simulink model "proj_sub"  (R2022b)
settings: Solver=VariableStepAuto  StartTime=0.0  StopTime=10.0  RelTol=1e-3
undefined symbols (not defined in the file): a, b, c, DiscIntNeverNeededParam
libraries: hdlsllib x6, slpidlib x4, dspswit3 x1
settings Model: Creator=fadii  LastModifiedBy=fadii

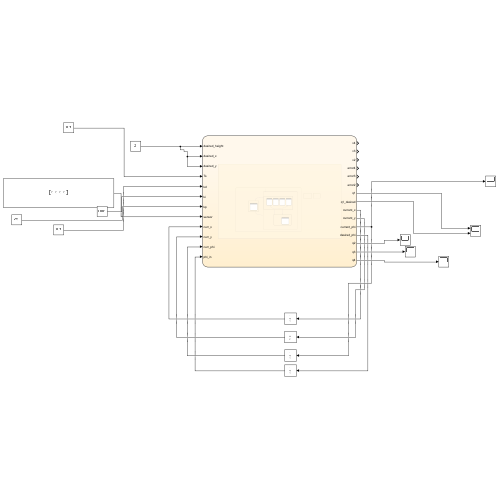
[thumbnail: Simulink's stored preview of the top-level diagram]
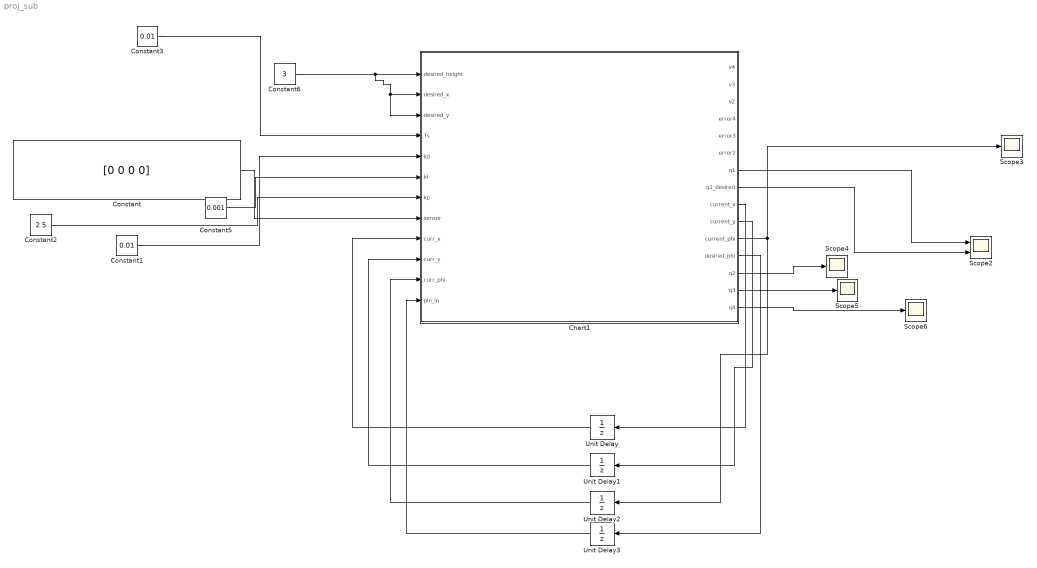
== system proj_sub ==
  Chart1 : Stateflow chart  TreatAsAtomicUnit=on
  Constant : Constant  Value=[0 0 0 0]
  Constant1 : Constant  Value=0.01
  Constant2 : Constant  Value=2.5
  Constant3 : Constant  Value=0.01
  Constant5 : Constant  Value=0.001
  Constant6 : Constant  Value=3
  Scope2 : Scope  NumInputPorts=2
  Scope{3..6} (4 alike) : Scope
  Unit Delay{,1..3} (4 alike) : UnitDelay  SampleTime=-1  HasFrameUpgradeWarning=on
  wires:
  Chart1/13(q2) -> Scope4/1
  Unit Delay1/1 -> Chart1/10(curr_y)
  Chart1/10(current_y) -> Unit Delay1/1
  Unit Delay2/1 -> Chart1/11(curr_phi)
  Constant6/1 -> Chart1/3(desired_y), Chart1/2(desired_x), Chart1/1(desired_height)
  Constant2/1 -> Chart1/7(kp)
  Constant3/1 -> Chart1/4(Ts)
  Chart1/14(q3) -> Scope5/1
  Chart1/12(desired_phi) -> Unit Delay3/1
  Chart1/11(current_phi) -> Scope3/1, Unit Delay2/1
  Chart1/8(q1_desired) -> Scope2/2
  Chart1/9(current_x) -> Unit Delay/1
  Constant1/1 -> Chart1/5(kd)
  Unit Delay3/1 -> Chart1/12(phi_in)
  Chart1/15(q4) -> Scope6/1
  Chart1/7(q1) -> Scope2/1
  Unit Delay/1 -> Chart1/9(curr_x)
  Constant/1 -> Chart1/8(sensor)
  Constant5/1 -> Chart1/6(ki)

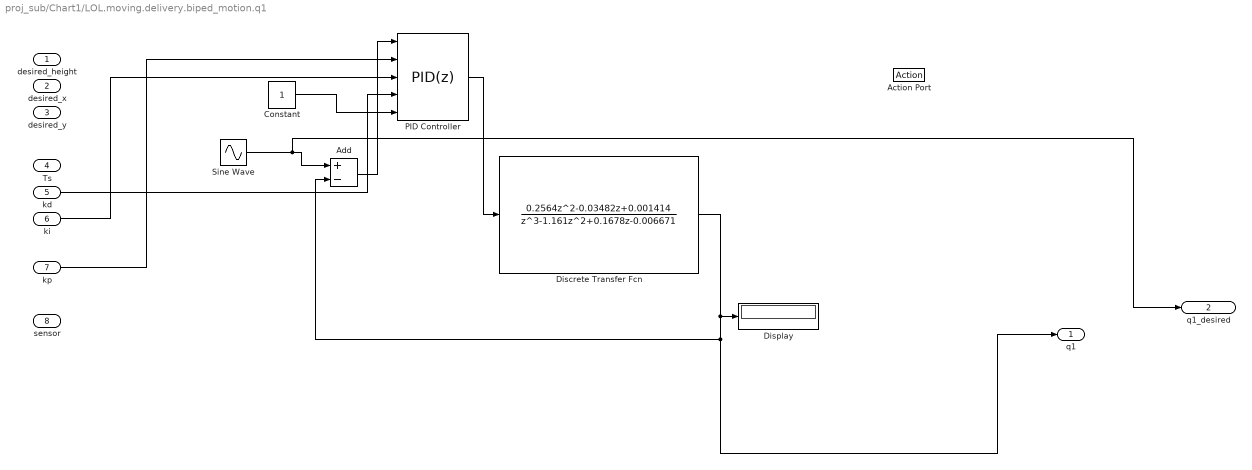
== system proj_sub/Chart1/LOL.moving.delivery.biped_motion.q1 ==
  desired_height : Inport
  desired_x : Inport  Port=2
  desired_y : Inport  Port=3
  Ts : Inport  Port=4
  kd : Inport  Port=5
  ki : Inport  Port=6
  kp : Inport  Port=7
  sensor : Inport  Port=8
  Action Port : ActionPort
      settings: CopyFcn=Stateflow.SLINSF.SimulinkMan.removeBlockPreDeleteFcn  PreDeleteFcn=Stateflow.SLINSF.SimulinkMan.unsafePredeleteFcn
  Add : Sum  Inputs=+-
  Constant : Constant
  Discrete Transfer Fcn : DiscreteTransferFcn  Numerator=[0 0.2564 -0.03482 0.001414]  Denominator=[1 -1.161 0.1678 -0.006671]  SampleTime=0.1
  Display : Display
  PID Controller : slpidlib/PID Controller  Controller=PID  Form=Parallel  TimeDomain=Discrete-time  UseExternalTs=off  SampleTime=0.1  IntegratorMethod=Forward Euler  FilterMethod=Forward Euler  ControllerParametersSource=external  P=1  I=0.002  UseKiTs=off  D=0.01  N=100  UseFilter=on  TunerSelectOption=Transfer Function Based (PID Tuner App)  InitialConditionSource=internal  InitialConditionForIntegrator=0  InitialConditionForFilter=0  DifferentiatorICPrevScaledInput=0  ExternalReset=none  TrackingMode=off  Kt=1  LimitOutput=on  SatLimitsSource=internal  UpperSaturationLimit=24  LowerSaturationLimit=-24  LinearizeAsGain=on  AntiWindupMode=none  Kb=1  LimitIntegrator=off  UpperIntegratorSaturationLimit=inf  LowerIntegratorSaturationLimit=-inf  POutMin=[]  POutMax=[]  IOutMin=[]  IOutMax=[]  DOutMin=[]  DOutMax=[]  NOutMin=[]  NOutMax=[]  SumOutMin=[]  SumOutMax=[]  SaturationOutMin=[]  SaturationOutMax=[]  PParamMin=[]  PParamMax=[]  IParamMin=[]  IParamMax=[]  DParamMin=[]  DParamMax=[]  NParamMin=[]  NParamMax=[]  KbParamMin=[]  KbParamMax=[]  KtParamMin=[]  KtParamMax=[]  KbOutMin=[]  KbOutMax=[]  KtOutMin=[]  KtOutMax=[]  IntegratorOutMin=[]  IntegratorOutMax=[]  FilterOutMin=[]  FilterOutMax=[]  SumI1OutMin=[]  SumI1OutMax=[]  SumI2OutMin=[]  SumI2OutMax=[]  SumI3OutMin=[]  SumI3OutMax=[]  SumI4OutMin=[]  SumI4OutMax=[]  SumDOutMin=[]  SumDOutMax=[]  DifferentiatorOutMin=[]  DifferentiatorOutMax=[]  FilterDiffOutCoefMin=[]  FilterDiffOutCoefMax=[]  ReciprocalOutMin=[]  ReciprocalOutMax=[]  SumDenOutMin=[]  SumDenOutMax=[]  SumNumOutMin=[]  SumNumOutMax=[]  DivideOutMin=[]  DivideOutMax=[]  UdiffTsProdOutMin=[]  UdiffTsProdOutMax=[]  NTsProdOutMin=[]  NTsProdOutMax=[]  UintegralTsProdOutMin=[]  UintegralTsProdOutMax=[]  UngainTsProdOutMin=[]  UngainTsProdOutMax=[]  ClampingZeroOutDataTypeStr=Inherit: Inherit via back propagation  ClampingZeroOutMin=[]  ClampingZeroOutMax=[]  FilterDenConstantOutDataTypeStr=Inherit: Inherit via back propagation  FilterDenConstantOutMin=[]  FilterDenConstantOutMax=[]  PCopyOutDataTypeStr=Inherit: Inherit via back propagation  PCopyOutMin=[]  PCopyOutMax=[]  NCopyOutDataTypeStr=Inherit: Inherit via back propagation  NCopyOutMin=[]  NCopyOutMax=[]  IntegratorContinuousStateAttributes=''  IntegratorStateMustResolveToSignalObject=off  IntegratorRTWStateStorageClass=Auto  FilterContinuousStateAttributes=''  FilterStateMustResolveToSignalObject=off  FilterRTWStateStorageClass=Auto  ParallelPVariant=ExternalParameters  IdealPVariant=Disabled  IVariant=ExternalParameters  DVariant=ExternalParameters  IntegratorVariant=Discrete  SatVariant=Enabled  AWVariant=Passthrough  PCopyVariant=Disabled  TRVariant=Disabled  FdbkBlocksVariant=Forward  IdealPFdbkVariant=Disabled  SatFdbkVariant=Disabled  DerivativeFilterVariant=ForwardEulerFilter  NVariant=ExternalParameters  NCopyVariant=Disabled  FilterICVariant=InternalICsFilter  IntegratorICVariant=InternalICs  ExternalResetVariant=Disabled  TRSumVariant=Passthrough  SumFdbkVariant=Disabled  SumVariant=Sum_PID  TsampFilterVariant=InternalTs  TsampNgainVariant=Passthrough  TsampIntegralVariant=Passthrough  ExternalSaturationOutDataTypeStr=Inherit: Same as second input
  Sine Wave : Sin  SineType=Sample based  Amplitude=20*pi/180  SampleTime=0.1
  q1 : Outport
  q1_desired : Outport  Port=2
  wires:
  Sine Wave/1 -> q1_desired/1, Add/1
  Add/1 -> PID Controller/1
  PID Controller/1 -> Discrete Transfer Fcn/1
  Discrete Transfer Fcn/1 -> q1/1, Add/2, Display/1
  Constant/1 -> PID Controller/5
  kp/1 -> PID Controller/2
  ki/1 -> PID Controller/3
  kd/1 -> PID Controller/4

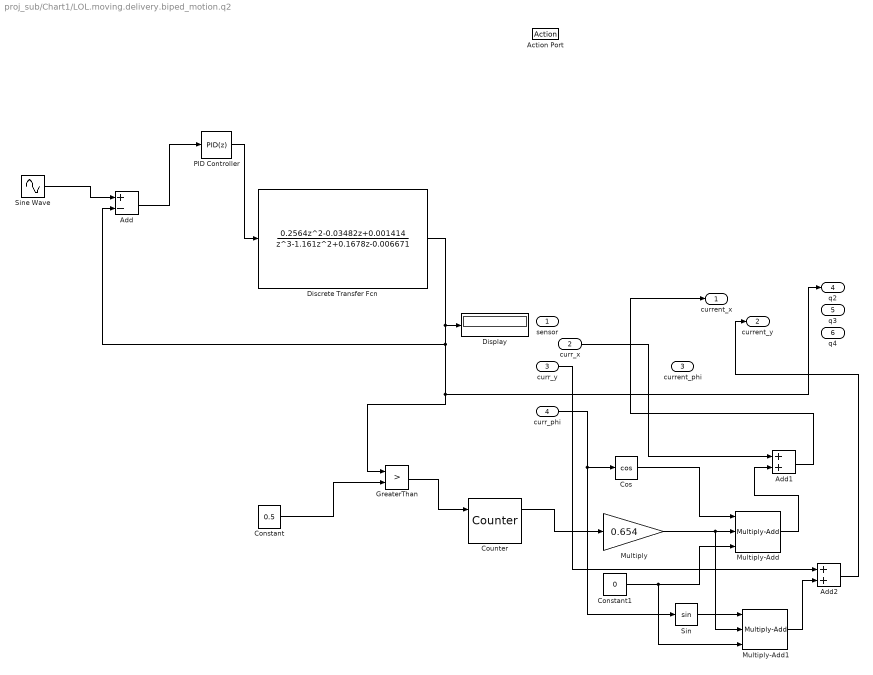
== system proj_sub/Chart1/LOL.moving.delivery.biped_motion.q2 ==
  sensor : Inport
  curr_x : Inport  Port=2
  curr_y : Inport  Port=3
  curr_phi : Inport  Port=4
  Action Port : ActionPort
      settings: CopyFcn=Stateflow.SLINSF.SimulinkMan.removeBlockPreDeleteFcn  PreDeleteFcn=Stateflow.SLINSF.SimulinkMan.unsafePredeleteFcn
  Add : Sum  Inputs=+-
  Add1 : Sum
  Add2 : Sum
  Constant : Constant  Value=0.5
  Constant1 : Constant  Value=0
  Cos : Trigonometry  Operator=cos
  Counter : dspswit3/Counter  Direction=Up  CountEvent=Rising edge  CounterSize=User defined  MaxCount=1024  InitialCount=0  Output=Count and Hit  HitValue=32  ResetInput=on  SamplesPerFrame=1  Ts=1  CntDtype=double  HitDtype=Logical
  Discrete Transfer Fcn : DiscreteTransferFcn  Numerator=[0 0.2564 -0.03482 0.001414]  Denominator=[1 -1.161 0.1678 -0.006671]  SampleTime=0.1
  Display : Display
  GreaterThan : RelationalOperator  Operator=>  OutDataTypeStr=boolean  RndMeth=Simplest  InputSameDT=off
  Multiply : Gain  Gain=0.654
  Multiply-Add : hdlsllib/HDL Operations/Multiply-Add  Function=c+(a.*b)  datatype=Inherit: Inherit via internal rule  DoSatur=off  FMA=off
  Multiply-Add1 : hdlsllib/HDL Operations/Multiply-Add  Function=c+(a.*b)  datatype=Inherit: Inherit via internal rule  DoSatur=off  FMA=off
  PID Controller : slpidlib/PID Controller  Controller=PID  Form=Parallel  TimeDomain=Discrete-time  UseExternalTs=off  SampleTime=0.1  IntegratorMethod=Forward Euler  FilterMethod=Forward Euler  ControllerParametersSource=internal  P=1  I=1  UseKiTs=off  D=0  N=100  UseFilter=on  TunerSelectOption=Transfer Function Based (PID Tuner App)  InitialConditionSource=internal  InitialConditionForIntegrator=0  InitialConditionForFilter=0  DifferentiatorICPrevScaledInput=0  ExternalReset=none  TrackingMode=off  Kt=1  LimitOutput=off  SatLimitsSource=internal  UpperSaturationLimit=inf  LowerSaturationLimit=-inf  LinearizeAsGain=on  AntiWindupMode=none  Kb=1  LimitIntegrator=off  UpperIntegratorSaturationLimit=inf  LowerIntegratorSaturationLimit=-inf  POutMin=[]  POutMax=[]  IOutMin=[]  IOutMax=[]  DOutMin=[]  DOutMax=[]  NOutMin=[]  NOutMax=[]  SumOutMin=[]  SumOutMax=[]  SaturationOutMin=[]  SaturationOutMax=[]  PParamMin=[]  PParamMax=[]  IParamMin=[]  IParamMax=[]  DParamMin=[]  DParamMax=[]  NParamMin=[]  NParamMax=[]  KbParamMin=[]  KbParamMax=[]  KtParamMin=[]  KtParamMax=[]  KbOutMin=[]  KbOutMax=[]  KtOutMin=[]  KtOutMax=[]  IntegratorOutMin=[]  IntegratorOutMax=[]  FilterOutMin=[]  FilterOutMax=[]  SumI1OutMin=[]  SumI1OutMax=[]  SumI2OutMin=[]  SumI2OutMax=[]  SumI3OutMin=[]  SumI3OutMax=[]  SumI4OutMin=[]  SumI4OutMax=[]  SumDOutMin=[]  SumDOutMax=[]  DifferentiatorOutMin=[]  DifferentiatorOutMax=[]  FilterDiffOutCoefMin=[]  FilterDiffOutCoefMax=[]  ReciprocalOutMin=[]  ReciprocalOutMax=[]  SumDenOutMin=[]  SumDenOutMax=[]  SumNumOutMin=[]  SumNumOutMax=[]  DivideOutMin=[]  DivideOutMax=[]  UdiffTsProdOutMin=[]  UdiffTsProdOutMax=[]  NTsProdOutMin=[]  NTsProdOutMax=[]  UintegralTsProdOutMin=[]  UintegralTsProdOutMax=[]  UngainTsProdOutMin=[]  UngainTsProdOutMax=[]  ClampingZeroOutDataTypeStr=Inherit: Inherit via back propagation  ClampingZeroOutMin=[]  ClampingZeroOutMax=[]  FilterDenConstantOutDataTypeStr=Inherit: Inherit via back propagation  FilterDenConstantOutMin=[]  FilterDenConstantOutMax=[]  PCopyOutDataTypeStr=Inherit: Inherit via back propagation  PCopyOutMin=[]  PCopyOutMax=[]  NCopyOutDataTypeStr=Inherit: Inherit via back propagation  NCopyOutMin=[]  NCopyOutMax=[]  IntegratorContinuousStateAttributes=''  IntegratorStateMustResolveToSignalObject=off  IntegratorRTWStateStorageClass=Auto  FilterContinuousStateAttributes=''  FilterStateMustResolveToSignalObject=off  FilterRTWStateStorageClass=Auto  ParallelPVariant=InternalParameters  IdealPVariant=Disabled  IVariant=InternalParameters  DVariant=InternalParameters  IntegratorVariant=Discrete  SatVariant=Disabled  AWVariant=Passthrough  PCopyVariant=Disabled  TRVariant=Disabled  FdbkBlocksVariant=Forward  IdealPFdbkVariant=Disabled  SatFdbkVariant=Disabled  DerivativeFilterVariant=ForwardEulerFilter  NVariant=InternalParameters  NCopyVariant=Disabled  FilterICVariant=InternalICsFilter  IntegratorICVariant=InternalICs  ExternalResetVariant=Disabled  TRSumVariant=Passthrough  SumFdbkVariant=Disabled  SumVariant=Sum_PID  TsampFilterVariant=InternalTs  TsampNgainVariant=Passthrough  TsampIntegralVariant=Passthrough  ExternalSaturationOutDataTypeStr=Inherit: Same as second input
  Sin : Trigonometry
  Sine Wave : Sin  SineType=Sample based  Amplitude=30*pi/180  Bias=30*pi/180  SampleTime=0.1  Offset=2
  current_x : Outport
  current_y : Outport  Port=2
  current_phi : Outport  Port=3
  q2 : Outport  Port=4
  q3 : Outport  Port=5
  q4 : Outport  Port=6
  wires:
  Constant/1 -> GreaterThan/2
  GreaterThan/1 -> Counter/1
  Add/1 -> PID Controller/1
  Discrete Transfer Fcn/1 -> GreaterThan/1, q2/1, Add/2, Display/1
  PID Controller/1 -> Discrete Transfer Fcn/1
  Sine Wave/1 -> Add/1
  Counter/1 -> Multiply/1
  curr_phi/1 -> Sin/1, Cos/1
  curr_x/1 -> Add1/1
  Add1/1 -> current_x/1
  Constant1/1 -> Multiply-Add1/3, Multiply-Add/3
  Multiply/1 -> Multiply-Add1/2, Multiply-Add/2
  Cos/1 -> Multiply-Add/1
  Multiply-Add/1 -> Add1/2
  Sin/1 -> Multiply-Add1/1
  Multiply-Add1/1 -> Add2/2
  curr_y/1 -> Add2/1
  Add2/1 -> current_y/1

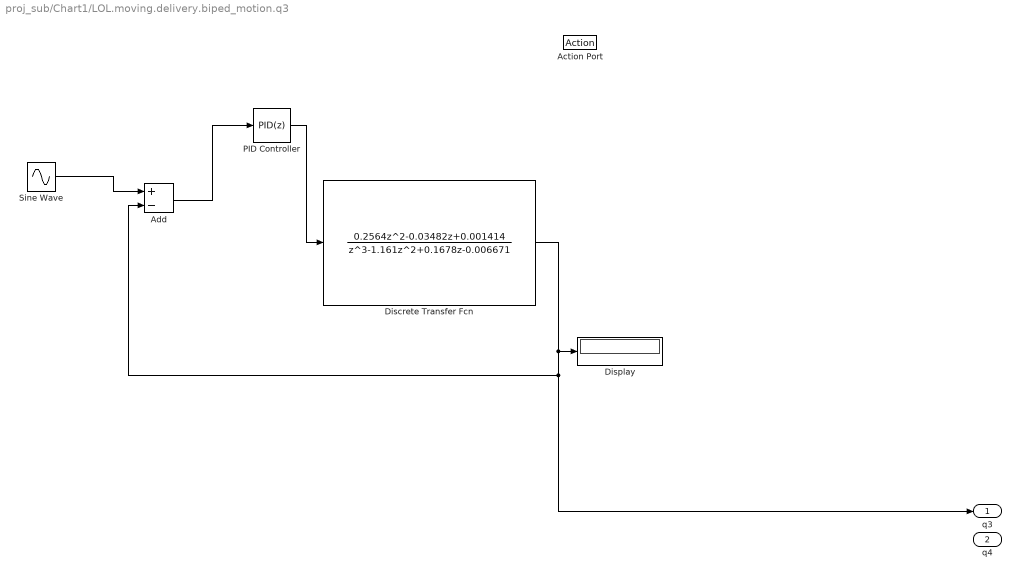
== system proj_sub/Chart1/LOL.moving.delivery.biped_motion.q3 ==
  Action Port : ActionPort
      settings: CopyFcn=Stateflow.SLINSF.SimulinkMan.removeBlockPreDeleteFcn  PreDeleteFcn=Stateflow.SLINSF.SimulinkMan.unsafePredeleteFcn
  Add : Sum  Inputs=+-
  Discrete Transfer Fcn : DiscreteTransferFcn  Numerator=[0 0.2564 -0.03482 0.001414]  Denominator=[1 -1.161 0.1678 -0.006671]  SampleTime=0.1
  Display : Display
  PID Controller : slpidlib/PID Controller  Controller=PID  Form=Parallel  TimeDomain=Discrete-time  UseExternalTs=off  SampleTime=0.1  IntegratorMethod=Forward Euler  FilterMethod=Forward Euler  ControllerParametersSource=internal  P=1  I=1  UseKiTs=off  D=0  N=100  UseFilter=on  TunerSelectOption=Transfer Function Based (PID Tuner App)  InitialConditionSource=internal  InitialConditionForIntegrator=0  InitialConditionForFilter=0  DifferentiatorICPrevScaledInput=0  ExternalReset=none  TrackingMode=off  Kt=1  LimitOutput=off  SatLimitsSource=internal  UpperSaturationLimit=inf  LowerSaturationLimit=-inf  LinearizeAsGain=on  AntiWindupMode=none  Kb=1  LimitIntegrator=off  UpperIntegratorSaturationLimit=inf  LowerIntegratorSaturationLimit=-inf  POutMin=[]  POutMax=[]  IOutMin=[]  IOutMax=[]  DOutMin=[]  DOutMax=[]  NOutMin=[]  NOutMax=[]  SumOutMin=[]  SumOutMax=[]  SaturationOutMin=[]  SaturationOutMax=[]  PParamMin=[]  PParamMax=[]  IParamMin=[]  IParamMax=[]  DParamMin=[]  DParamMax=[]  NParamMin=[]  NParamMax=[]  KbParamMin=[]  KbParamMax=[]  KtParamMin=[]  KtParamMax=[]  KbOutMin=[]  KbOutMax=[]  KtOutMin=[]  KtOutMax=[]  IntegratorOutMin=[]  IntegratorOutMax=[]  FilterOutMin=[]  FilterOutMax=[]  SumI1OutMin=[]  SumI1OutMax=[]  SumI2OutMin=[]  SumI2OutMax=[]  SumI3OutMin=[]  SumI3OutMax=[]  SumI4OutMin=[]  SumI4OutMax=[]  SumDOutMin=[]  SumDOutMax=[]  DifferentiatorOutMin=[]  DifferentiatorOutMax=[]  FilterDiffOutCoefMin=[]  FilterDiffOutCoefMax=[]  ReciprocalOutMin=[]  ReciprocalOutMax=[]  SumDenOutMin=[]  SumDenOutMax=[]  SumNumOutMin=[]  SumNumOutMax=[]  DivideOutMin=[]  DivideOutMax=[]  UdiffTsProdOutMin=[]  UdiffTsProdOutMax=[]  NTsProdOutMin=[]  NTsProdOutMax=[]  UintegralTsProdOutMin=[]  UintegralTsProdOutMax=[]  UngainTsProdOutMin=[]  UngainTsProdOutMax=[]  ClampingZeroOutDataTypeStr=Inherit: Inherit via back propagation  ClampingZeroOutMin=[]  ClampingZeroOutMax=[]  FilterDenConstantOutDataTypeStr=Inherit: Inherit via back propagation  FilterDenConstantOutMin=[]  FilterDenConstantOutMax=[]  PCopyOutDataTypeStr=Inherit: Inherit via back propagation  PCopyOutMin=[]  PCopyOutMax=[]  NCopyOutDataTypeStr=Inherit: Inherit via back propagation  NCopyOutMin=[]  NCopyOutMax=[]  IntegratorContinuousStateAttributes=''  IntegratorStateMustResolveToSignalObject=off  IntegratorRTWStateStorageClass=Auto  FilterContinuousStateAttributes=''  FilterStateMustResolveToSignalObject=off  FilterRTWStateStorageClass=Auto  ParallelPVariant=InternalParameters  IdealPVariant=Disabled  IVariant=InternalParameters  DVariant=InternalParameters  IntegratorVariant=Discrete  SatVariant=Disabled  AWVariant=Passthrough  PCopyVariant=Disabled  TRVariant=Disabled  FdbkBlocksVariant=Forward  IdealPFdbkVariant=Disabled  SatFdbkVariant=Disabled  DerivativeFilterVariant=ForwardEulerFilter  NVariant=InternalParameters  NCopyVariant=Disabled  FilterICVariant=InternalICsFilter  IntegratorICVariant=InternalICs  ExternalResetVariant=Disabled  TRSumVariant=Passthrough  SumFdbkVariant=Disabled  SumVariant=Sum_PID  TsampFilterVariant=InternalTs  TsampNgainVariant=Passthrough  TsampIntegralVariant=Passthrough  ExternalSaturationOutDataTypeStr=Inherit: Same as second input
  Sine Wave : Sin  SineType=Sample based  Amplitude=20*pi/180  SampleTime=0.1  Offset=10
  q3 : Outport
  q4 : Outport  Port=2
  wires:
  Sine Wave/1 -> Add/1
  Add/1 -> PID Controller/1
  PID Controller/1 -> Discrete Transfer Fcn/1
  Discrete Transfer Fcn/1 -> q3/1, Add/2, Display/1

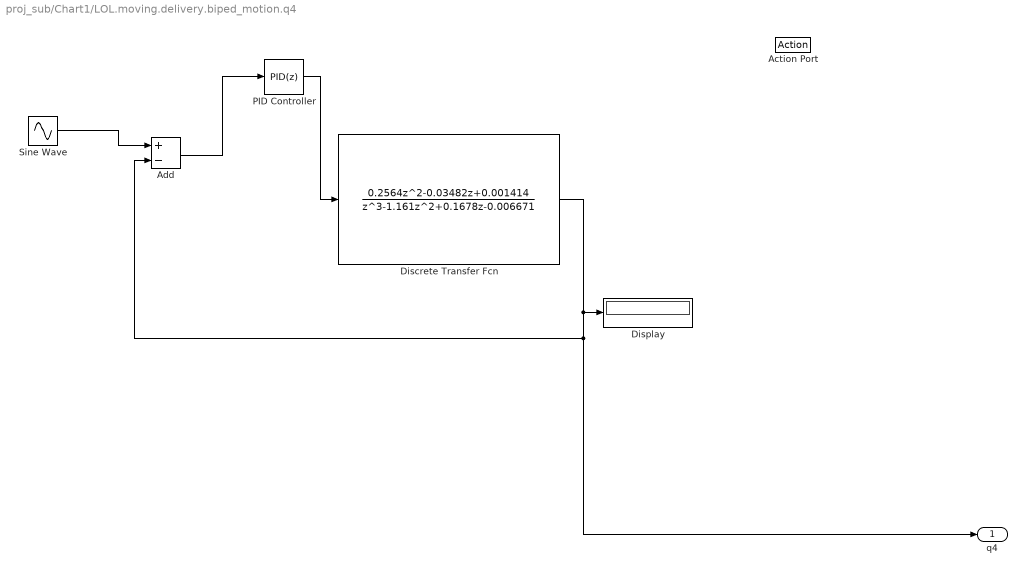
== system proj_sub/Chart1/LOL.moving.delivery.biped_motion.q4 ==
  Action Port : ActionPort
      settings: CopyFcn=Stateflow.SLINSF.SimulinkMan.removeBlockPreDeleteFcn  PreDeleteFcn=Stateflow.SLINSF.SimulinkMan.unsafePredeleteFcn
  Add : Sum  Inputs=+-
  Discrete Transfer Fcn : DiscreteTransferFcn  Numerator=[0 0.2564 -0.03482 0.001414]  Denominator=[1 -1.161 0.1678 -0.006671]  SampleTime=0.1
  Display : Display
  PID Controller : slpidlib/PID Controller  Controller=PID  Form=Parallel  TimeDomain=Discrete-time  UseExternalTs=off  SampleTime=0.1  IntegratorMethod=Forward Euler  FilterMethod=Forward Euler  ControllerParametersSource=internal  P=1  I=1  UseKiTs=off  D=0  N=100  UseFilter=on  TunerSelectOption=Transfer Function Based (PID Tuner App)  InitialConditionSource=internal  InitialConditionForIntegrator=0  InitialConditionForFilter=0  DifferentiatorICPrevScaledInput=0  ExternalReset=none  TrackingMode=off  Kt=1  LimitOutput=off  SatLimitsSource=internal  UpperSaturationLimit=inf  LowerSaturationLimit=-inf  LinearizeAsGain=on  AntiWindupMode=none  Kb=1  LimitIntegrator=off  UpperIntegratorSaturationLimit=inf  LowerIntegratorSaturationLimit=-inf  POutMin=[]  POutMax=[]  IOutMin=[]  IOutMax=[]  DOutMin=[]  DOutMax=[]  NOutMin=[]  NOutMax=[]  SumOutMin=[]  SumOutMax=[]  SaturationOutMin=[]  SaturationOutMax=[]  PParamMin=[]  PParamMax=[]  IParamMin=[]  IParamMax=[]  DParamMin=[]  DParamMax=[]  NParamMin=[]  NParamMax=[]  KbParamMin=[]  KbParamMax=[]  KtParamMin=[]  KtParamMax=[]  KbOutMin=[]  KbOutMax=[]  KtOutMin=[]  KtOutMax=[]  IntegratorOutMin=[]  IntegratorOutMax=[]  FilterOutMin=[]  FilterOutMax=[]  SumI1OutMin=[]  SumI1OutMax=[]  SumI2OutMin=[]  SumI2OutMax=[]  SumI3OutMin=[]  SumI3OutMax=[]  SumI4OutMin=[]  SumI4OutMax=[]  SumDOutMin=[]  SumDOutMax=[]  DifferentiatorOutMin=[]  DifferentiatorOutMax=[]  FilterDiffOutCoefMin=[]  FilterDiffOutCoefMax=[]  ReciprocalOutMin=[]  ReciprocalOutMax=[]  SumDenOutMin=[]  SumDenOutMax=[]  SumNumOutMin=[]  SumNumOutMax=[]  DivideOutMin=[]  DivideOutMax=[]  UdiffTsProdOutMin=[]  UdiffTsProdOutMax=[]  NTsProdOutMin=[]  NTsProdOutMax=[]  UintegralTsProdOutMin=[]  UintegralTsProdOutMax=[]  UngainTsProdOutMin=[]  UngainTsProdOutMax=[]  ClampingZeroOutDataTypeStr=Inherit: Inherit via back propagation  ClampingZeroOutMin=[]  ClampingZeroOutMax=[]  FilterDenConstantOutDataTypeStr=Inherit: Inherit via back propagation  FilterDenConstantOutMin=[]  FilterDenConstantOutMax=[]  PCopyOutDataTypeStr=Inherit: Inherit via back propagation  PCopyOutMin=[]  PCopyOutMax=[]  NCopyOutDataTypeStr=Inherit: Inherit via back propagation  NCopyOutMin=[]  NCopyOutMax=[]  IntegratorContinuousStateAttributes=''  IntegratorStateMustResolveToSignalObject=off  IntegratorRTWStateStorageClass=Auto  FilterContinuousStateAttributes=''  FilterStateMustResolveToSignalObject=off  FilterRTWStateStorageClass=Auto  ParallelPVariant=InternalParameters  IdealPVariant=Disabled  IVariant=InternalParameters  DVariant=InternalParameters  IntegratorVariant=Discrete  SatVariant=Disabled  AWVariant=Passthrough  PCopyVariant=Disabled  TRVariant=Disabled  FdbkBlocksVariant=Forward  IdealPFdbkVariant=Disabled  SatFdbkVariant=Disabled  DerivativeFilterVariant=ForwardEulerFilter  NVariant=InternalParameters  NCopyVariant=Disabled  FilterICVariant=InternalICsFilter  IntegratorICVariant=InternalICs  ExternalResetVariant=Disabled  TRSumVariant=Passthrough  SumFdbkVariant=Disabled  SumVariant=Sum_PID  TsampFilterVariant=InternalTs  TsampNgainVariant=Passthrough  TsampIntegralVariant=Passthrough  ExternalSaturationOutDataTypeStr=Inherit: Same as second input
  Sine Wave : Sin  SineType=Sample based  Amplitude=30*pi/180  SampleTime=0.1  Offset=12
  q4 : Outport
  wires:
  Sine Wave/1 -> Add/1
  Add/1 -> PID Controller/1
  PID Controller/1 -> Discrete Transfer Fcn/1
  Discrete Transfer Fcn/1 -> q4/1, Add/2, Display/1

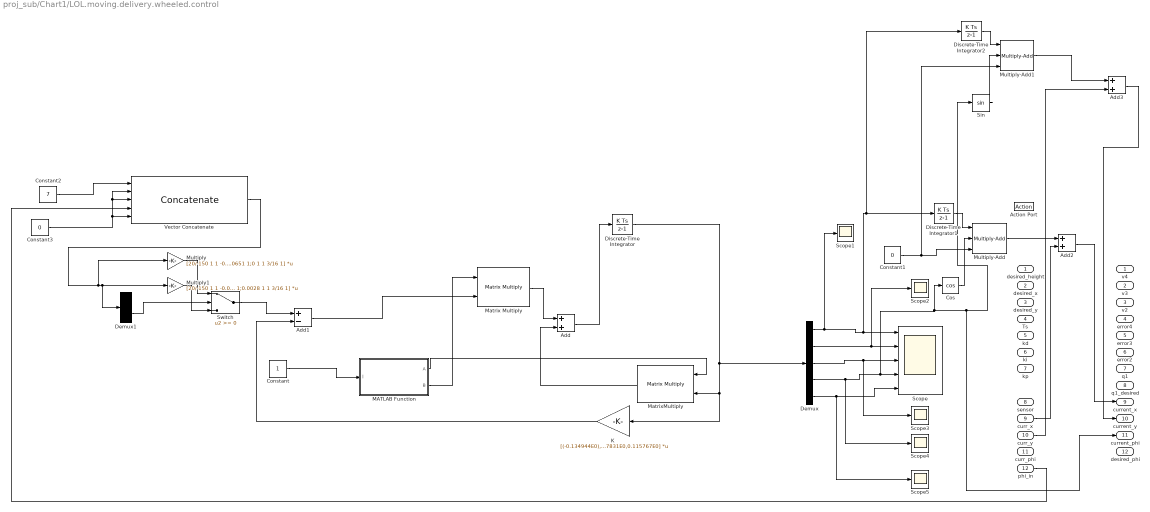
== system proj_sub/Chart1/LOL.moving.delivery.wheeled.control ==
  desired_height : Inport
  desired_x : Inport  Port=2
  desired_y : Inport  Port=3
  Ts : Inport  Port=4
  kd : Inport  Port=5
  ki : Inport  Port=6
  kp : Inport  Port=7
  sensor : Inport  Port=8
  curr_x : Inport  Port=9
  curr_y : Inport  Port=10
  curr_phi : Inport  Port=11
  phi_in : Inport  Port=12
  Action Port : ActionPort
      settings: CopyFcn=Stateflow.SLINSF.SimulinkMan.removeBlockPreDeleteFcn  PreDeleteFcn=Stateflow.SLINSF.SimulinkMan.unsafePredeleteFcn
  Add : Sum
  Add1 : Sum  Inputs=+-
  Add2 : Sum
  Add3 : Sum
  Constant : Constant
  Constant1 : Constant  Value=0
  Constant2 : Constant  Value=7
  Constant3 : Constant  Value=0
  Cos : Trigonometry  Operator=cos
  Demux : Demux  Outputs=5
  Demux1 : Demux  Outputs=5
  Discrete-Time Integrator : DiscreteIntegrator  SampleTime=-1  ICPrevOutput=DiscIntNeverNeededParam  ICPrevScaledInput=DiscIntNeverNeededParam
  Discrete-Time Integrator1 : DiscreteIntegrator  SampleTime=-1  ICPrevOutput=DiscIntNeverNeededParam  ICPrevScaledInput=DiscIntNeverNeededParam
  Discrete-Time Integrator2 : DiscreteIntegrator  SampleTime=-1  ICPrevOutput=DiscIntNeverNeededParam  ICPrevScaledInput=DiscIntNeverNeededParam
  K : Gain  Gain=[(-0.134944E0),(-0.371525E1),(-0.913882E0),(-0.137452E0),(-0.125089E0);0.90514E-3,(-0.273949E1),(-0.607007E0),0.177831E0,0.115767E0]  Multiplication=Matrix(K*u)
  MATLAB Function : MATLAB Function  TreatAsAtomicUnit=on
  Matrix Multiply : Product  Multiplication=Matrix(*)
  MatrixMultiply : Product  Multiplication=Matrix(*)
  Multiply : Gain  Gain=[20/-150 1 1 -0.0651 1;0 1 1 3/16 1]  Multiplication=Matrix(K*u)
  Multiply-Add : hdlsllib/HDL Operations/Multiply-Add  Function=c+(a.*b)  datatype=Inherit: Inherit via internal rule  DoSatur=off  FMA=off
  Multiply-Add1 : hdlsllib/HDL Operations/Multiply-Add  Function=c+(a.*b)  datatype=Inherit: Inherit via internal rule  DoSatur=off  FMA=off
  Multiply1 : Gain  Gain=[20/-150 1 1 -0.0681 1;0.0028 1 1 3/16 1]  Multiplication=Matrix(K*u)
  Scope : Scope  NumInputPorts=5
  Scope{1..5} (5 alike) : Scope
  Sin : Trigonometry
  Switch : Switch  SaturateOnIntegerOverflow=off  InputSameDT=off
  Vector Concatenate : Concatenate  NumInputs=5
  v4 : Outport
  v3 : Outport  Port=2
  v2 : Outport  Port=3
  error4 : Outport  Port=4
  error3 : Outport  Port=5
  error2 : Outport  Port=6
  q1 : Outport  Port=7
  q1_desired : Outport  Port=8
  current_x : Outport  Port=9
  current_y : Outport  Port=10
  current_phi : Outport  Port=11
  desired_phi : Outport  Port=12
  wires:
  Multiply/1 -> Switch/1
  Vector Concatenate/1 -> Multiply/1, Multiply1/1, Demux1/1
  Demux1/4 -> Switch/2
  Switch/1 -> Add1/1
  Multiply1/1 -> Switch/3
  Discrete-Time Integrator/1 -> K/1, MatrixMultiply/2, Demux/1
  K/1 -> Add1/2
  Demux/3 -> Scope3/1, Scope/3
  MATLAB Function/2(B) -> Matrix Multiply/1
  Matrix Multiply/1 -> Add/1
  Constant/1 -> MATLAB Function/1(l)
  Add/1 -> Discrete-Time Integrator/1
  MATLAB Function/1(A) -> MatrixMultiply/1
  MatrixMultiply/1 -> Add/2
  Add1/1 -> Matrix Multiply/2
  Demux/2 -> Scope2/1, Scope/2
  Demux/5 -> Scope5/1, Scope/5
  Constant2/1 -> Vector Concatenate/1
  Constant3/1 -> Vector Concatenate/5, Vector Concatenate/3, Vector Concatenate/2
  phi_in/1 -> Vector Concatenate/4
  Cos/1 -> Multiply-Add/2
  Discrete-Time Integrator1/1 -> Multiply-Add/1
  Multiply-Add/1 -> Add2/1
  curr_x/1 -> Add2/2
  Add2/1 -> current_x/1
  Discrete-Time Integrator2/1 -> Multiply-Add1/1
  Demux/4 -> Scope4/1, current_phi/1, Sin/1, Cos/1, Scope/4
  Constant1/1 -> Multiply-Add1/3, Multiply-Add/3
  Sin/1 -> Multiply-Add1/2
  Demux/1 -> Discrete-Time Integrator2/1, Discrete-Time Integrator1/1, Scope/1, Scope1/1
  Multiply-Add1/1 -> Add3/1
  curr_y/1 -> Add3/2
  Add3/1 -> current_y/1

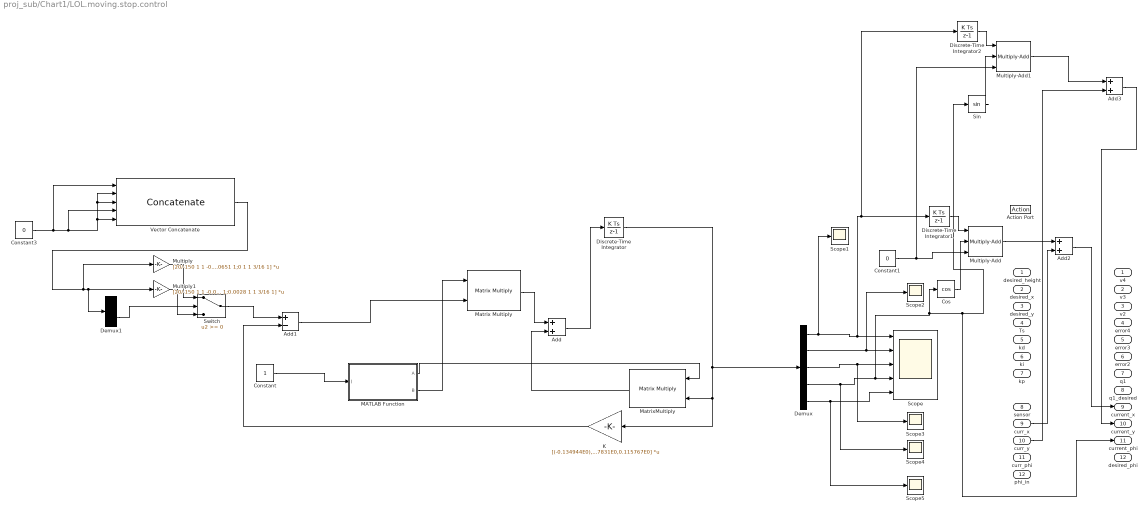
== system proj_sub/Chart1/LOL.moving.stop.control ==
  desired_height : Inport
  desired_x : Inport  Port=2
  desired_y : Inport  Port=3
  Ts : Inport  Port=4
  kd : Inport  Port=5
  ki : Inport  Port=6
  kp : Inport  Port=7
  sensor : Inport  Port=8
  curr_x : Inport  Port=9
  curr_y : Inport  Port=10
  curr_phi : Inport  Port=11
  phi_in : Inport  Port=12
  Action Port : ActionPort
      settings: CopyFcn=Stateflow.SLINSF.SimulinkMan.removeBlockPreDeleteFcn  PreDeleteFcn=Stateflow.SLINSF.SimulinkMan.unsafePredeleteFcn
  Add : Sum
  Add1 : Sum  Inputs=+-
  Add2 : Sum
  Add3 : Sum
  Constant : Constant
  Constant1 : Constant  Value=0
  Constant3 : Constant  Value=0
  Cos : Trigonometry  Operator=cos
  Demux : Demux  Outputs=5
  Demux1 : Demux  Outputs=5
  Discrete-Time Integrator : DiscreteIntegrator  SampleTime=-1  ICPrevOutput=DiscIntNeverNeededParam  ICPrevScaledInput=DiscIntNeverNeededParam
  Discrete-Time Integrator1 : DiscreteIntegrator  SampleTime=-1  ICPrevOutput=DiscIntNeverNeededParam  ICPrevScaledInput=DiscIntNeverNeededParam
  Discrete-Time Integrator2 : DiscreteIntegrator  SampleTime=-1  ICPrevOutput=DiscIntNeverNeededParam  ICPrevScaledInput=DiscIntNeverNeededParam
  K : Gain  Gain=[(-0.134944E0),(-0.371525E1),(-0.913882E0),(-0.137452E0),(-0.125089E0);0.90514E-3,(-0.273949E1),(-0.607007E0),0.177831E0,0.115767E0]  Multiplication=Matrix(K*u)
  MATLAB Function : MATLAB Function  TreatAsAtomicUnit=on
  Matrix Multiply : Product  Multiplication=Matrix(*)
  MatrixMultiply : Product  Multiplication=Matrix(*)
  Multiply : Gain  Gain=[20/-150 1 1 -0.0651 1;0 1 1 3/16 1]  Multiplication=Matrix(K*u)
  Multiply-Add : hdlsllib/HDL Operations/Multiply-Add  Function=c+(a.*b)  datatype=Inherit: Inherit via internal rule  DoSatur=off  FMA=off
  Multiply-Add1 : hdlsllib/HDL Operations/Multiply-Add  Function=c+(a.*b)  datatype=Inherit: Inherit via internal rule  DoSatur=off  FMA=off
  Multiply1 : Gain  Gain=[20/-150 1 1 -0.0681 1;0.0028 1 1 3/16 1]  Multiplication=Matrix(K*u)
  Scope : Scope  NumInputPorts=5
  Scope{1..5} (5 alike) : Scope
  Sin : Trigonometry
  Switch : Switch  SaturateOnIntegerOverflow=off  InputSameDT=off
  Vector Concatenate : Concatenate  NumInputs=5
  v4 : Outport
  v3 : Outport  Port=2
  v2 : Outport  Port=3
  error4 : Outport  Port=4
  error3 : Outport  Port=5
  error2 : Outport  Port=6
  q1 : Outport  Port=7
  q1_desired : Outport  Port=8
  current_x : Outport  Port=9
  current_y : Outport  Port=10
  current_phi : Outport  Port=11
  desired_phi : Outport  Port=12
  wires:
  Multiply/1 -> Switch/1
  Vector Concatenate/1 -> Multiply/1, Multiply1/1, Demux1/1
  Demux1/4 -> Switch/2
  Switch/1 -> Add1/1
  Multiply1/1 -> Switch/3
  Discrete-Time Integrator/1 -> K/1, MatrixMultiply/2, Demux/1
  K/1 -> Add1/2
  Demux/3 -> Scope3/1, Scope/3
  MATLAB Function/2(B) -> Matrix Multiply/1
  Matrix Multiply/1 -> Add/1
  Constant/1 -> MATLAB Function/1(l)
  Add/1 -> Discrete-Time Integrator/1
  MATLAB Function/1(A) -> MatrixMultiply/1
  MatrixMultiply/1 -> Add/2
  Add1/1 -> Matrix Multiply/2
  Demux/2 -> Scope2/1, Scope/2
  Demux/5 -> Scope5/1, Scope/5
  Constant3/1 -> Vector Concatenate/1, Vector Concatenate/4, Vector Concatenate/5, Vector Concatenate/3, Vector Concatenate/2
  Cos/1 -> Multiply-Add/2
  Discrete-Time Integrator1/1 -> Multiply-Add/1
  Multiply-Add/1 -> Add2/1
  curr_x/1 -> Add2/2
  Add2/1 -> current_x/1
  Discrete-Time Integrator2/1 -> Multiply-Add1/1
  Demux/4 -> Scope4/1, current_phi/1, Sin/1, Cos/1, Scope/4
  Constant1/1 -> Multiply-Add1/3, Multiply-Add/3
  Sin/1 -> Multiply-Add1/2
  Demux/1 -> Discrete-Time Integrator2/1, Discrete-Time Integrator1/1, Scope/1, Scope1/1
  Multiply-Add1/1 -> Add3/1
  curr_y/1 -> Add3/2
  Add3/1 -> current_y/1

== matlab function proj_sub/Chart1/LOL.moving.stop.control/MATLAB Function ==
  data: l input; A output; B output
function [A,B]= get_A_B(l)
Mw = 0.5;
r = 0.2;
m = 1;
M = 1;
Iw = 0.00375;
Ip = 0.00631;
Ix = 0.0261;
d = 0.45;
g = 9.81;
A=[0,g.*l.*m.*(Ip+2.*d.^2.*(Mw+Iw.*r.^(-2))).^(-1).*((-1).*Ip.*l.*M+ ...
(-2).*d.^2.*l.*M.*Mw+(-2).*d.^2.*Iw.*l.*M.*r.^(-2)).*(Ix.*M+2.* ...
Ix.*Mw+2.*l.^2.*M.*Mw+2.*Iw.*Ix.*r.^(-2)+2.*Iw.*l.^2.*M.*r.^(-2)) ...
.^(-1),0,0,0;0,0,1,0,0;0,g.*l.*m.*(M+2.*Mw+2.*Iw.*r.^(-2)).*(Ix.* ...
M+2.*Ix.*Mw+2.*l.^2.*M.*Mw+2.*Iw.*Ix.*r.^(-2)+2.*Iw.*l.^2.*M.*r.^( ...
-2)).^(-1),0,0,0;0,0,0,0,(-1).*((-1).*Ix.*M+(-2).*Ix.*Mw+(-2).* ...
l.^2.*M.*Mw+(-2).*Iw.*Ix.*r.^(-2)+(-2).*Iw.*l.^2.*M.*r.^(-2)).*( ...
Ix.*M+2.*Ix.*Mw+2.*l.^2.*M.*Mw+2.*Iw.*Ix.*r.^(-2)+2.*Iw.*l.^2.*M.* ...
r.^(-2)).^(-1);0,0,0,0,0];
B=[(Ix+l.^2.*M).*(Ip+2.*d.^2.*(Mw+Iw.*r.^(-2))).^(-1).*(Ip+2.*d.^2.* ...
Mw+2.*d.^2.*Iw.*r.^(-2)).*(Ix.*M+2.*Ix.*Mw+2.*l.^2.*M.*Mw+2.*Iw.* ...
Ix.*r.^(-2)+2.*Iw.*l.^2.*M.*r.^(-2)).^(-1).*r.^(-1),(Ix+l.^2.*M).* ...
(Ip+2.*d.^2.*(Mw+Iw.*r.^(-2))).^(-1).*(Ip+2.*d.^2.*Mw+2.*d.^2.* ...
Iw.*r.^(-2)).*(Ix.*M+2.*Ix.*Mw+2.*l.^2.*M.*Mw+2.*Iw.*Ix.*r.^(-2)+ ...
2.*Iw.*l.^2.*M.*r.^(-2)).^(-1).*r.^(-1);0,0;(Ip+2.*d.^2.*(Mw+Iw.* ...
r.^(-2))).^(-1).*((-1).*Ip.*l.*M+(-2).*d.^2.*l.*M.*Mw+(-2).*d.^2.* ...
Iw.*l.*M.*r.^(-2)).*(Ix.*M+2.*Ix.*Mw+2.*l.^2.*M.*Mw+2.*Iw.*Ix.* ...
r.^(-2)+2.*Iw.*l.^2.*M.*r.^(-2)).^(-1).*r.^(-1),(Ip+2.*d.^2.*(Mw+ ...
Iw.*r.^(-2))).^(-1).*((-1).*Ip.*l.*M+(-2).*d.^2.*l.*M.*Mw+(-2).* ...
d.^2.*Iw.*l.*M.*r.^(-2)).*(Ix.*M+2.*Ix.*Mw+2.*l.^2.*M.*Mw+2.*Iw.* ...
Ix.*r.^(-2)+2.*Iw.*l.^2.*M.*r.^(-2)).^(-1).*r.^(-1);0,0;(-2).*d.*( ...
Ip+2.*d.^2.*(Mw+Iw.*r.^(-2))).^(-1).*r.^(-1),2.*d.*(Ip+2.*d.^2.*( ...
Mw+Iw.*r.^(-2))).^(-1).*r.^(-1)];
end

== stateflow chart proj_sub/Chart1 ==
  state LOL
    state moving [parallel]
      settings: executionOrder=1
      state delivery
        state biped_motion
          entry:
          state q1
          state q2
          state q3
          state q4
          (default) -> q1
          q1 -> q2 : [after(100,msec)]
          q3 -> q4 : [after(300,msec)]
          q2 -> q3 : [after(200,msec)]
          q4 -> q1 : [after(400,msec)]
        state wheeled
          state control
          (default) -> LOL.moving.delivery.wheeled.control
        wheeled -> biped_motion : [tough_terrain==1]
        biped_motion -> wheeled : [tough_terrain==0]
        (default) -> wheeled
      state stop
        state control
        (default) -> LOL.moving.stop.control
      (default) -> delivery
      delivery -> stop : [path_achieved == 1]
      stop -> delivery : [path_achieved == 0]
    state obstact_detector [parallel]
      entry:
      positions = sensor
      if sum(positions,'all')>30
      tough_terrain=1
      else
      tough_terrain=0
      flag=0
      end
      settings: executionOrder=2
    state Path_checker [parallel]
      entry:
      if abs(curr_x-desired_x) <1
      if abs(curr_y-desired_y) <1
      path_achieved=1
      end
      else
      path_achieved=0;
      end
      settings: executionOrder=3
  data: sf_internal_action_state_placeholder_data local double size=1 =0; sf_internal_action_state_placeholder_data local double size=1 =0; sf_internal_action_state_placeholder_data local double size=1 =0; sf_internal_action_state_placeholder_data local double size=1 =0; sf_internal_action_state_placeholder_data local double size=1 =0; sf_internal_action_state_placeholder_data local double size=1 =0; desired_height input; desired_x input; desired_y input; Ts input; kd input; ki input; kp input; tough_terrain local; positions local; v4 output =0; v3 output =0; v2 output =0; error4 output =0; error3 output =0; error2 output =0; sensor input; q1 output =0; flag local =1; q1_desired output =0; curr_x input; curr_y input; curr_phi input; current_x output =0; current_y output =0; current_phi output =0; desired_phi output =0; phi_in input; q2 output =0; q3 output =0; q4 output =0; path_achieved local

== matlab function proj_sub/Chart1/LOL.moving.delivery.wheeled.control/MATLAB Function ==
  data: l input; A output; B output
function [A,B]= get_A_B(l)
Mw = 0.5;
r = 0.2;
m = 1;
M = 1;
Iw = 0.00375;
Ip = 0.00631;
Ix = 0.0261;
d = 0.45;
g = 9.81;
A=[0,g.*l.*m.*(Ip+2.*d.^2.*(Mw+Iw.*r.^(-2))).^(-1).*((-1).*Ip.*l.*M+ ...
(-2).*d.^2.*l.*M.*Mw+(-2).*d.^2.*Iw.*l.*M.*r.^(-2)).*(Ix.*M+2.* ...
Ix.*Mw+2.*l.^2.*M.*Mw+2.*Iw.*Ix.*r.^(-2)+2.*Iw.*l.^2.*M.*r.^(-2)) ...
.^(-1),0,0,0;0,0,1,0,0;0,g.*l.*m.*(M+2.*Mw+2.*Iw.*r.^(-2)).*(Ix.* ...
M+2.*Ix.*Mw+2.*l.^2.*M.*Mw+2.*Iw.*Ix.*r.^(-2)+2.*Iw.*l.^2.*M.*r.^( ...
-2)).^(-1),0,0,0;0,0,0,0,(-1).*((-1).*Ix.*M+(-2).*Ix.*Mw+(-2).* ...
l.^2.*M.*Mw+(-2).*Iw.*Ix.*r.^(-2)+(-2).*Iw.*l.^2.*M.*r.^(-2)).*( ...
Ix.*M+2.*Ix.*Mw+2.*l.^2.*M.*Mw+2.*Iw.*Ix.*r.^(-2)+2.*Iw.*l.^2.*M.* ...
r.^(-2)).^(-1);0,0,0,0,0];
B=[(Ix+l.^2.*M).*(Ip+2.*d.^2.*(Mw+Iw.*r.^(-2))).^(-1).*(Ip+2.*d.^2.* ...
Mw+2.*d.^2.*Iw.*r.^(-2)).*(Ix.*M+2.*Ix.*Mw+2.*l.^2.*M.*Mw+2.*Iw.* ...
Ix.*r.^(-2)+2.*Iw.*l.^2.*M.*r.^(-2)).^(-1).*r.^(-1),(Ix+l.^2.*M).* ...
(Ip+2.*d.^2.*(Mw+Iw.*r.^(-2))).^(-1).*(Ip+2.*d.^2.*Mw+2.*d.^2.* ...
Iw.*r.^(-2)).*(Ix.*M+2.*Ix.*Mw+2.*l.^2.*M.*Mw+2.*Iw.*Ix.*r.^(-2)+ ...
2.*Iw.*l.^2.*M.*r.^(-2)).^(-1).*r.^(-1);0,0;(Ip+2.*d.^2.*(Mw+Iw.* ...
r.^(-2))).^(-1).*((-1).*Ip.*l.*M+(-2).*d.^2.*l.*M.*Mw+(-2).*d.^2.* ...
Iw.*l.*M.*r.^(-2)).*(Ix.*M+2.*Ix.*Mw+2.*l.^2.*M.*Mw+2.*Iw.*Ix.* ...
r.^(-2)+2.*Iw.*l.^2.*M.*r.^(-2)).^(-1).*r.^(-1),(Ip+2.*d.^2.*(Mw+ ...
Iw.*r.^(-2))).^(-1).*((-1).*Ip.*l.*M+(-2).*d.^2.*l.*M.*Mw+(-2).* ...
d.^2.*Iw.*l.*M.*r.^(-2)).*(Ix.*M+2.*Ix.*Mw+2.*l.^2.*M.*Mw+2.*Iw.* ...
Ix.*r.^(-2)+2.*Iw.*l.^2.*M.*r.^(-2)).^(-1).*r.^(-1);0,0;(-2).*d.*( ...
Ip+2.*d.^2.*(Mw+Iw.*r.^(-2))).^(-1).*r.^(-1),2.*d.*(Ip+2.*d.^2.*( ...
Mw+Iw.*r.^(-2))).^(-1).*r.^(-1)];
end
